simulink model "ITK_VTKModel"  (Simulink 6.6)
settings: Solver=FixedStepDiscrete  StartTime=0.0  StopTime=inf  FixedStep=0.1  RelTol=1e-3
libraries: SimITKLibraryFL2D x2, SimvtkImagingLibrary x2, SimvtkRenderingLibrary x1, SimvtkCommonLibrary x1
settings Model: Creator=dgobbi  LastModifiedBy=dgobbi

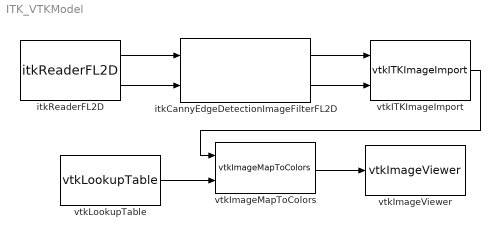
== system ITK_VTKModel ==
  itkCannyEdgeDetectionImageFilterFL2D : SimITKLibraryFL2D/itkCannyEdgeDetectionImageFilterFL2D  LowerThreshold=10  MaximumError=[0.01 0.01]  OutsideValue=0  UpperThreshold=30  Variance=[0.1 0.1]
  itkReaderFL2D : SimITKLibraryFL2D/itkReaderFL2D  FileName='cthead1.png'
  vtkITKImageImport : SimvtkImagingLibrary/vtkITKImageImport  dataType=Float
  vtkImageMapToColors : SimvtkImagingLibrary/vtkImageMapToColors  VTKInputSelf=off  VTKInputLookupTable=on  ActiveComponentInputIndicator=Use Default  VTKParamActiveComponent=0  NumberOfThreadsInputIndicator=Use Default  VTKParamNumberOfThreads=0  NumberOfThreadsMaxValueInputIndicator=off  VTKParamNumberOfThreadsMaxValue=0  NumberOfThreadsMinValueInputIndicator=off  VTKParamNumberOfThreadsMinValue=0  OutputFormatInputIndicator=Use Default  VTKParamOutputFormat=0  PassAlphaToOutputInputIndicator=Use Default  VTKParamPassAlphaToOutput=0  VTKOutputSelf=off
  vtkImageViewer : SimvtkRenderingLibrary/vtkImageViewer  VTKInputSelf=off  VTKInputInput=on  VTKInputInputConnection=off  VTKInputupInteractor=off  ColorLevelInputIndicator=As Parameter  VTKParamColorLevel=127.5  ColorWindowInputIndicator=As Parameter  VTKParamColorWindow=255  GrayScaleHintInputIndicator=Use Default  VTKParamGrayScaleHint=0  OffScreenRenderingInputIndicator=Use Default  VTKParamOffScreenRendering=0  PositionInputIndicator=Use Default  VTKParamPosition=[0,0]  SizeInputIndicator=Use Default  VTKParamSize=[0,0]  WholeZMaxInputIndicator=off  VTKParamWholeZMax=0  WholeZMinInputIndicator=off  VTKParamWholeZMin=0  WindowNameInputIndicator=off  VTKParamWindowName=0  ZSliceInputIndicator=Use Default  VTKParamZSlice=0  VTKOutputSelf=off  VTKOutputActor2D=off  VTKOutputImageMapper=off  VTKOutputRenderWindow=off  VTKOutputRenderer=off
  vtkLookupTable : SimvtkCommonLibrary/vtkLookupTable  VTKInputSelf=off  VTKInputTable=off  AlphaInputIndicator=Use Default  VTKParamAlpha=0  AlphaRangeInputIndicator=Use Default  VTKParamAlphaRange=[0,0]  HueRangeInputIndicator=Use Default  VTKParamHueRange=[0,0]  RampInputIndicator=Use Default  VTKParamRamp=0  RangeInputIndicator=As Parameter  VTKParamRange=[0, 1]  SaturationRangeInputIndicator=As Parameter  VTKParamSaturationRange=[0,0]  ScaleInputIndicator=Use Default  VTKParamScale=0  TableRangeInputIndicator=Use Default  VTKParamTableRange=[0,0]  ValueRangeInputIndicator=As Parameter  VTKParamValueRange=[0,1]  VectorComponentInputIndicator=Use Default  VTKParamVectorComponent=0  VectorModeInputIndicator=Use Default  VTKParamVectorMode=0  VTKOutputSelf=on
  wires:
  vtkLookupTable/1 -> vtkImageMapToColors/2
  vtkImageMapToColors/1 -> vtkImageViewer/1
  itkReaderFL2D/1 -> itkCannyEdgeDetectionImageFilterFL2D/1
  itkReaderFL2D/2 -> itkCannyEdgeDetectionImageFilterFL2D/2
  itkCannyEdgeDetectionImageFilterFL2D/1 -> vtkITKImageImport/1
  itkCannyEdgeDetectionImageFilterFL2D/2 -> vtkITKImageImport/2
  vtkITKImageImport/1 -> vtkImageMapToColors/1
